simulink model "task3_1_Lyapunov"  (R2023a)
settings: Solver=VariableStepAuto  StartTime=0.0  StopTime=100  RelTol=1e-3
settings Model: Creator=10366  LastModifiedBy=10366

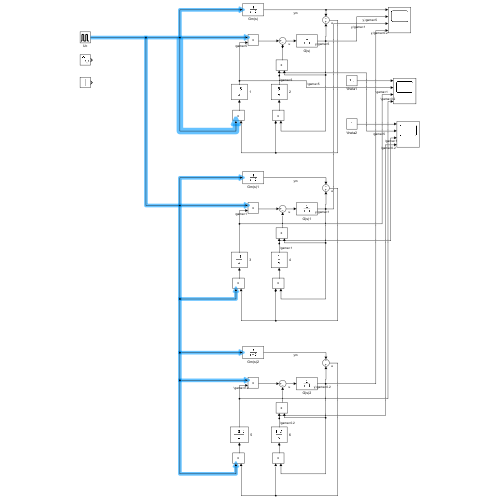
[thumbnail: Simulink's stored preview of the top-level diagram]
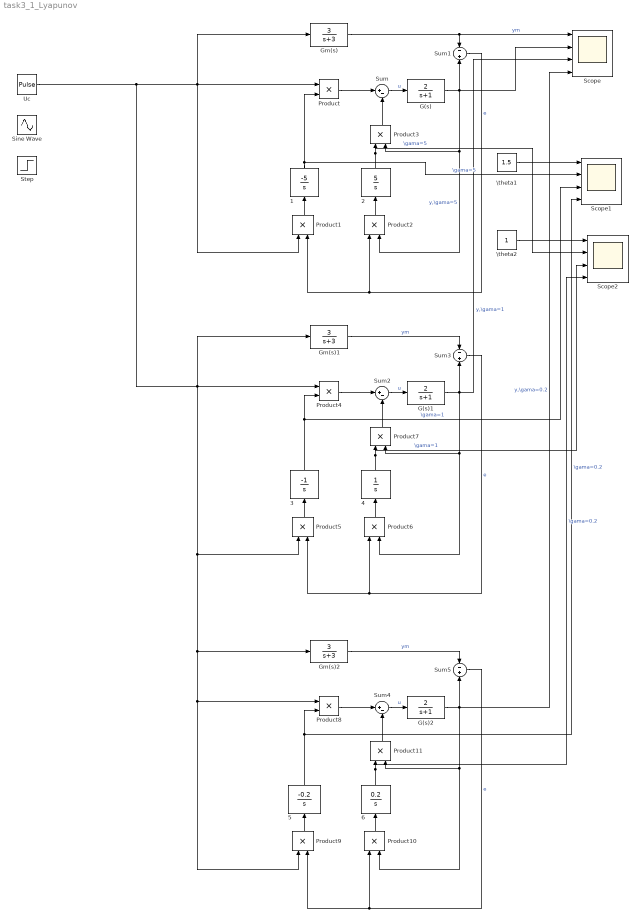
== system task3_1_Lyapunov ==
  1 : TransferFcn  Numerator=[-5]  Denominator=[1 0]
  2 : TransferFcn  Numerator=[5]  Denominator=[1 0]
  3 : TransferFcn  Numerator=[-1]  Denominator=[1 0]
  4 : TransferFcn  Denominator=[1 0]
  5 : TransferFcn  Numerator=[-0.2]  Denominator=[1 0]
  6 : TransferFcn  Numerator=[0.2]  Denominator=[1 0]
  G(s) : TransferFcn  Numerator=[2]  Denominator=[1 1]
  G(s)1 : TransferFcn  Numerator=[2]  Denominator=[1 1]
  G(s)2 : TransferFcn  Numerator=[2]  Denominator=[1 1]
  Gm(s) : TransferFcn  Numerator=[3]  Denominator=[1 3]
  Gm(s)1 : TransferFcn  Numerator=[3]  Denominator=[1 3]
  Gm(s)2 : TransferFcn  Numerator=[3]  Denominator=[1 3]
  Product{,1..11} (12 alike) : Product
  Scope : Scope  NumInputPorts=4
  Scope1 : Scope  NumInputPorts=4
  Scope2 : Scope  NumInputPorts=4
  Sine Wave : Sin  Amplitude=2  Frequency=0.4  SampleTime=0
  Step : Step  Time=0  After=2  SampleTime=0
  Sum : Sum  Inputs=|+-
  Sum1 : Sum  Inputs=-|+
  Sum2 : Sum  Inputs=|+-
  Sum3 : Sum  Inputs=-|+
  Sum4 : Sum  Inputs=|+-
  Sum5 : Sum  Inputs=-|+
  Uc : DiscretePulseGenerator  PulseType=Time based  Amplitude=2  Period=10  PulseWidth=50
  \theta1 : Constant  Value=1.5
  \theta2 : Constant
  wires:
  Product1/1 -> 1/1
  1/1 -> Scope1/2, Product/2  "\\gama=5"
  Product/1 -> Sum/1
  Sum/1 -> G(s)/1  "u"
  G(s)/1 -> Scope/2, Sum1/2, Product2/2, Product3/2  "y,\\gama=5"
  Gm(s)/1 -> Sum1/1, Scope/1  "ym"
  Sum1/1 -> Product1/2, Product2/1  "e"
  Product2/1 -> 2/1
  2/1 -> Scope2/2, Product3/1  "\\gama=5"
  Product3/1 -> Sum/2
  Sum2/1 -> G(s)1/1  "u"
  G(s)1/1 -> Scope/3, Sum3/2, Product6/2, Product7/2  "y,\\gama=1"
  Sum3/1 -> Product5/2, Product6/1  "e"
  3/1 -> Scope1/3, Product4/2  "\\gama=1"
  Gm(s)1/1 -> Sum3/1  "ym"
  Product4/1 -> Sum2/1
  4/1 -> Scope2/3, Product7/1  "\\gama=1"
  Product5/1 -> 3/1
  Product7/1 -> Sum2/2
  Product6/1 -> 4/1
  Sum4/1 -> G(s)2/1  "u"
  G(s)2/1 -> Scope/4, Sum5/2, Product10/2, Product11/2  "y,\\gama=0.2"
  Uc/1 -> Product5/1, Product9/1, Product8/1, Gm(s)2/1, Product4/1, Gm(s)1/1, Product1/1, Product/1, Gm(s)/1
  Sum5/1 -> Product9/2, Product10/1  "e"
  5/1 -> Scope1/4, Product8/2  "\\gama=0.2"
  Gm(s)2/1 -> Sum5/1  "ym"
  Product8/1 -> Sum4/1
  6/1 -> Scope2/4, Product11/1  "\\gama=0.2"
  Product9/1 -> 5/1
  Product11/1 -> Sum4/2
  Product10/1 -> 6/1
  \theta1/1 -> Scope1/1
  \theta2/1 -> Scope2/1
